simulink model "TransferFxnMatch"  (R2021b)
settings: Solver=VariableStepAuto  StartTime=0.0  StopTime=1  RelTol=1e-3
values from neighbouring files (symbols this model uses):
  K = 11.5/255    (= 0.0450980392157)    [TxferMatch.m]
  sig = 13    [TxferMatch.m]
settings Model: Creator=conno  LastModifiedBy=conno

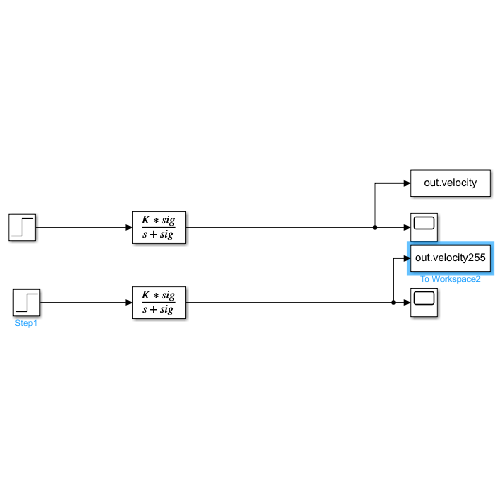
[thumbnail: Simulink's stored preview of the top-level diagram]
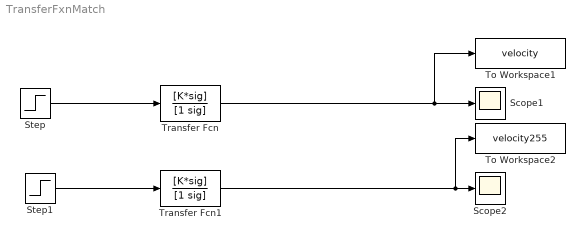
== system TransferFxnMatch ==
  Scope1 : Scope
  Scope2 : Scope
  Step : Step  Time=0.04  After=128  SampleTime=0
  Step1 : Step  Time=0.04  After=255  SampleTime=0
  To Workspace1 : ToWorkspace  VariableName=velocity  SaveFormat=Timeseries  SampleTime=-1
  To Workspace2 : ToWorkspace  VariableName=velocity255  SaveFormat=Timeseries  SampleTime=-1
  Transfer Fcn : TransferFcn  Numerator=[K*sig]  Denominator=[1 sig]
  Transfer Fcn1 : TransferFcn  Numerator=[K*sig]  Denominator=[1 sig]
  wires:
  Step/1 -> Transfer Fcn/1
  Transfer Fcn1/1 -> To Workspace2/1, Scope2/1
  Step1/1 -> Transfer Fcn1/1
  Transfer Fcn/1 -> To Workspace1/1, Scope1/1
